simulink model "question_vi_r2017b"  (R2022b)
settings: Solver=VariableStepAuto  StartTime=0.0  StopTime=10  RelTol=1e-3
values from neighbouring files (symbols this model uses):
  param =     [param.mat]
settings Model: Creator=15043  LastModifiedBy=15043
settings SolverCC: AlgebraicLoopSolver=TrustRegion
settings DebuggingCC: ArithmeticOperatorsInVariantConditions=warning
settings SFSimCC: CustomCodeUndefinedFunction=UseInterfaceOnly

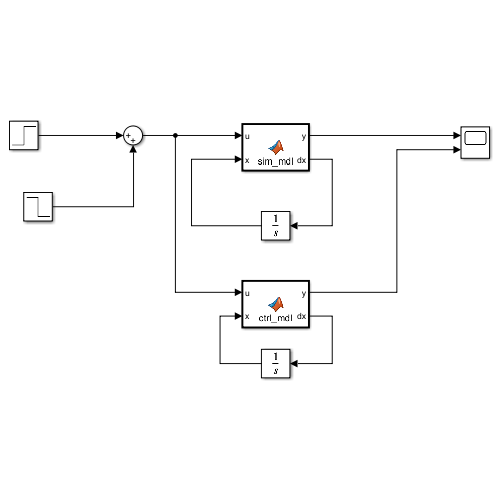
[thumbnail: Simulink's stored preview of the top-level diagram]
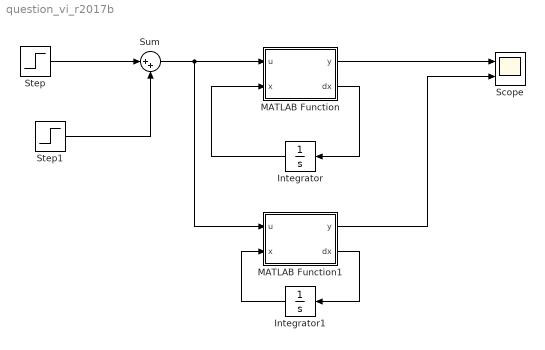
== system question_vi_r2017b ==
  Integrator : Integrator  InitialCondition=param.x0
  Integrator1 : Integrator  InitialCondition=param.x0
  MATLAB Function : MATLAB Function  TreatAsAtomicUnit=on
  MATLAB Function1 : MATLAB Function  TreatAsAtomicUnit=on
  Scope : Scope  NumInputPorts=2
  Step : Step  After=5  SampleTime=0
  Step1 : Step  Time=1.2  After=-5  SampleTime=0
  Sum : Sum  Inputs=|++
  wires:
  Step1/1 -> Sum/2
  Step/1 -> Sum/1
  MATLAB Function/2(dx) -> Integrator/1
  Integrator/1 -> MATLAB Function/2(x)
  Sum/1 -> MATLAB Function1/1(u), MATLAB Function/1(u)
  MATLAB Function/1(y) -> Scope/1
  MATLAB Function1/2(dx) -> Integrator1/1
  Integrator1/1 -> MATLAB Function1/2(x)
  MATLAB Function1/1(y) -> Scope/2

== matlab function question_vi_r2017b/MATLAB Function1 ==
  data: y output; dx output; u input; x input; param parameter
function [y, dx]= ctrl_mdl(u, x, param)

    g = param.g;
%     l_c = param.l_c;
%     l_ax = param.l_ax;
%     l_ay = param.l_ay;
%     k_f = param.k_t;
%     s_0 = param.s_0;
    k_r = 0.001;
    m_B1 = param.m_B1;
    m_B2 = param.m_B2;
%     l_B1 = param.l_B1;
%     l_B2 = param.l_B2;
    J_Pzz = param.J_Pzz;
    d_P = param.d_P;
    R_m = param.R_m;
    k_b = param.k_b;
    k_m = param.k_m;
    K_g = param.K_g;
    eta_g = param.eta_g;
    eta_m = param.eta_m;
    %nu = param.nu;
    J_Bzz = 0.00341;
    l_G = 0.172;


    x1 = x(1);
    x2 = x(2);
    x3 = x(3);
    x4 = x(4);
    
    f1 = x2;
    f3 = x4;
    f2 = (-(R_m*d_P + K_g*eta_g*eta_m*k_b*k_m)/(J_Pzz*R_m))*x2 + (k_r/J_Pzz)*x3;
    f4 = ((g*l_G*(m_B1 + m_B2))/J_Bzz)*sin(x1 + x3) + (x2*(R_m*d_P + K_g*eta_g*eta_m*k_b*k_m))/(J_Pzz*R_m) - (k_r*x3*(J_Bzz + J_Pzz))/(J_Bzz*J_Pzz);

    f = [f1; f2; f3; f4];
    
    g = [0;
        (K_g*eta_g*eta_m*k_b)/(J_Pzz*R_m);
        0;
        -(K_g*eta_g*eta_m*k_b)/(J_Pzz*R_m)];
    
    dx = f + g*u;
    y = x1 + x3;

end

== matlab function question_vi_r2017b/MATLAB Function ==
  data: y output; dx output; u input; x input; param parameter
function [y, dx]= sim_mdl(u, x, param)

    g = param.g;
    l_c = param.l_c;
    l_ax = param.l_ax;
    l_ay = param.l_ay;
    k_f = param.k_t;
    s_0 = param.s_0;
    m_B1 = param.m_B1;
    m_B2 = param.m_B2;
%     l_B1 = param.l_B1;
%     l_B2 = param.l_B2;
    J_Pzz = param.J_Pzz;
    d_P = param.d_P;
    R_m = param.R_m;
    k_b = param.k_b;
    k_m = param.k_m;
    K_g = param.K_g;
    eta_g = param.eta_g;
    eta_m = param.eta_m;
    %nu = param.nu;
    J_Bzz = 0.00341;
    l_G = 0.172;


    x1 = x(1);
    x2 = x(2);
    x3 = x(3);
    x4 = x(4);
    
    f1 = x2;
    f3 = x4;
    f2 =  (-((k_f*l_ax*l_c*s_0)/((l_ax - l_c*cos(x3))^2 + (l_ay + l_c*sin(x3))^2)^(1/2) - 2*k_f*l_ax*l_c + (k_f*l_ax*l_c*s_0)/((l_ax - l_c*cos(x3))^2 + (l_ay - l_c*sin(x3))^2)^(1/2))/J_Pzz)*sin(x3) + (-((k_f*l_ay*l_c*s_0)/((l_ax - l_c*cos(x3))^2 + (l_ay + l_c*sin(x3))^2)^(1/2) - (k_f*l_ay*l_c*s_0)/((l_ax - l_c*cos(x3))^2 + (l_ay - l_c*sin(x3))^2)^(1/2))/J_Pzz)*cos(x3) + (-(d_P + (K_g*eta_g*eta_m*k_b*k_m)/R_m)/J_Pzz)*x2;
    f4 =  ((g*l_G*m_B1 + g*l_G*m_B2)/J_Bzz)*sin(x1 + x3) + (((J_Bzz*((k_f*l_ax*l_c*s_0)/((l_ax - l_c*cos(x3))^2 + (l_ay + l_c*sin(x3))^2)^(1/2) - 2*k_f*l_ax*l_c + (k_f*l_ax*l_c*s_0)/((l_ax - l_c*cos(x3))^2 + (l_ay - l_c*sin(x3))^2)^(1/2)))/J_Pzz - 2*k_f*l_ax*l_c + (k_f*l_ax*l_c*s_0)/((l_ax - l_c*cos(x3))^2 + (l_ay + l_c*sin(x3))^2)^(1/2) + (k_f*l_ax*l_c*s_0)/((l_ax - l_c*cos(x3))^2 + (l_ay - l_c*sin(x3))^2)^(1/2))/J_Bzz)*sin(x3) + (((J_Bzz*((k_f*l_ay*l_c*s_0)/((l_ax - l_c*cos(x3))^2 + (l_ay + l_c*sin(x3))^2)^(1/2) - (k_f*l_ay*l_c*s_0)/((l_ax - l_c*cos(x3))^2 + (l_ay - l_c*sin(x3))^2)^(1/2)))/J_Pzz + (k_f*l_ay*l_c*s_0)/((l_ax - l_c*cos(x3))^2 + (l_ay + l_c*sin(x3))^2)^(1/2) - (k_f*l_ay*l_c*s_0)/((l_ax - l_c*cos(x3))^2 + (l_ay - l_c*sin(x3))^2)^(1/2))/J_Bzz)*cos(x3) + (d_P*x2 + (K_g*eta_g*eta_m*k_b*k_m*x2)/R_m)/J_Pzz;

    f = [f1; f2; f3; f4];
    
    g = [0;
        (K_g*eta_g*eta_m*k_b)/(J_Pzz*R_m);
        0;
        -(K_g*eta_g*eta_m*k_b)/(J_Pzz*R_m)];
    
    dx = f + g*u;
    y = x1 + x3;

end
